simulink model "test_three_phase_NPC_converter"  (R2017b)
settings: Solver=ode8  StartTime=0.0  StopTime=0.04  FixedStep=1e-6  MaxStep=1e-4  RelTol=1e-3
libraries: powerlib x9, typhoonHILlib x1
settings Model: Creator=Marcos  LastModifiedBy=Marcos

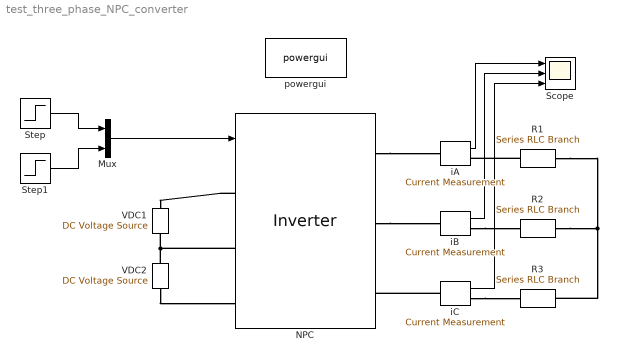
== system test_three_phase_NPC_converter ==
  Mux : Mux  Inputs=2
  NPC : typhoonHILlib/Inverter  InvType=NPC  ThreePhase=on  sa1_logic=Active-high  sa2_logic=Active-high  sa3_logic=Active-high  sa4_logic=Active-high  sa5_logic=Active-high  sa6_logic=Active-high  sb1_logic=Active-high  sb2_logic=Active-high  sb3_logic=Active-high  sb4_logic=Active-high  sb5_logic=Active-high  sb6_logic=Active-high  sc1_logic=Active-high  sc2_logic=Active-high  sc3_logic=Active-high  sc4_logic=Active-high  sc5_logic=Active-high  sc6_logic=Active-high  di_sa1=1  di_sa2=2  di_sa3=3  di_sa4=4  di_sa5=5  di_sa6=6  di_sb1=7  di_sb2=8  di_sb3=9  di_sb4=10  di_sb5=11  di_sb6=12  di_sc1=13  di_sc2=14  di_sc3=15  di_sc4=16  di_sc5=17  di_sc6=18  v_sa1=off  v_sa2=off  v_sa3=off  v_sa4=off  v_sa5=off  v_sa6=off  v_sb1=off  v_sb2=off  v_sb3=off  v_sb4=off  v_sb5=off  v_sb6=off  v_sc1=off  v_sc2=off  v_sc3=off  v_sc4=off  v_sc5=off  v_sc6=off  i_sa1=off  i_sa2=off  i_sa3=off  i_sa4=off  i_sa5=off  i_sa6=off  i_sb1=off  i_sb2=off  i_sb3=off  i_sb4=off  i_sb5=off  i_sb6=off  i_sc1=off  i_sc2=off  i_sc3=off  i_sc4=off  i_sc5=off  i_sc6=off  c_clamp=1e-6  v0_clamp=0  r_clamp=1e-4  r_on=0.001  v_f=0  r_s=1e4  c_s=inf  toggle_init=on  toggle_draw=on  model_loaded=off  old_pat=typhoonPatterns/NPC Inverter  old_size=140,215
      settings: SourceProductName=Typhoon HIL
  R1 : powerlib/Elements/Series RLC Branch  LConnTagsString=__new0  RConnTagsString=__new0  BranchType=R  Resistance=10  Inductance=1e-3  SetiL0=off  InitialCurrent=0  Capacitance=1e-6  Setx0=off  InitialVoltage=0  Measurements=None
  R2 : powerlib/Elements/Series RLC Branch  LConnTagsString=__new0  RConnTagsString=__new0  BranchType=R  Resistance=10  Inductance=1e-3  SetiL0=off  InitialCurrent=0  Capacitance=1e-6  Setx0=off  InitialVoltage=0  Measurements=None
  R3 : powerlib/Elements/Series RLC Branch  LConnTagsString=__new0  RConnTagsString=__new0  BranchType=R  Resistance=10  Inductance=1e-3  SetiL0=off  InitialCurrent=0  Capacitance=1e-6  Setx0=off  InitialVoltage=0  Measurements=None
  Scope : Scope  NumInputPorts=3
  Step : Step  Time=0.01  Before=[0 0 0 0 0 0 0 0 0 0]  After=[1 1 0 0 0 0 1 1 0 0]  SampleTime=0
  Step1 : Step  Time=0.02  Before=[0 0]  After=[1 1]  SampleTime=0
  VDC1 : powerlib/Electrical Sources/DC Voltage Source  Amplitude=75  Measurements=None
  VDC2 : powerlib/Electrical Sources/DC Voltage Source  Amplitude=75  Measurements=None
  iA : powerlib/Measurements/Current Measurement  PhasorSimulation=off  OutputType=Complex  PSBequivalent=0
  iB : powerlib/Measurements/Current Measurement  PhasorSimulation=off  OutputType=Complex  PSBequivalent=0
  iC : powerlib/Measurements/Current Measurement  PhasorSimulation=off  OutputType=Complex  PSBequivalent=0
  powergui : powerlib/powergui  Priority=1  SimulationMode=Discrete  SampleTime=1e-6  frequency=60  Iterations=50  frequencyindice=0  Pbase=100e6  ErrMax=1e-4  UnitsV=kV  UnitsW=MW  buscounter=0  FunctionMessages=off  echomessages=off  EnableUseOfTLC=off  CurrentSourceSwitches=off  DisableSnubberDevices=off  DisableRonSwitches=off  DisableVfSwitches=off  DisplayEquations=off  SolverType=Tustin/Backward Euler (TBE)  Interpol=off  ExternalGateDelay=off  methode=off  Ts=100  x0status=blocks  SPID=on  SwTol=0  HookPort=off  RestoreLinks=warning  ResistiveCurrentMeasurement=off  Frange=[0:2:500]  Ylog=off  Xlog=on  ShowGrid=off  save=off  variable=ZData  structure=0  ZoomFFT=off  StartTime=0.0  cycles=1  DisplayStyle=1  fundamental=60  FreqAxis=off  MaxFrequency=1000  frequencyindicesteady=1  RmsSteady=1  display=off
  wires:
  Mux/1 -> NPC/1
  Step/1 -> Mux/1
  Step1/1 -> Mux/2
  iA/1 -> Scope/1
  iB/1 -> Scope/2
  iC/1 -> Scope/3
  connections:
  R1/LConn1 -- iA/RConn1
  NPC/RConn1 -- iA/LConn1
  R1/RConn1 -- R2/RConn1 -- R3/RConn1
  NPC/LConn1 -- VDC1/RConn1
  VDC2/LConn1 -- NPC/LConn3
  VDC2/RConn1 -- NPC/LConn2 -- VDC1/LConn1
  iC/LConn1 -- NPC/RConn3
  NPC/RConn2 -- iB/LConn1
  iB/RConn1 -- R2/LConn1
  iC/RConn1 -- R3/LConn1
